simulink model "MohammadDBZ1"  (R2023b)
settings: Solver=ode15s  StartTime=0.0  StopTime=300  RelTol=1e-3
libraries: slpidlib x10
settings Model: PacingRate=10  Creator=Nezam Avaran  LastModifiedBy=Nezam Avaran

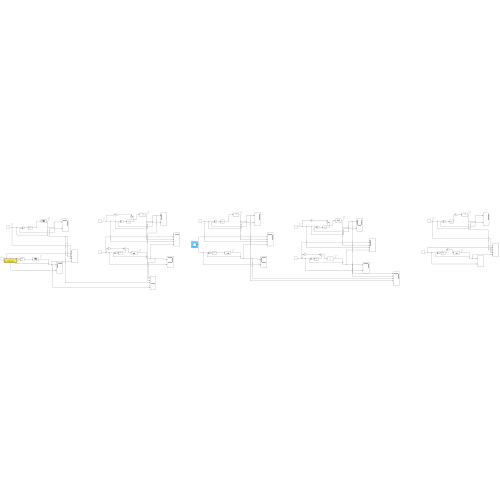
[thumbnail: Simulink's stored preview of the top-level diagram]
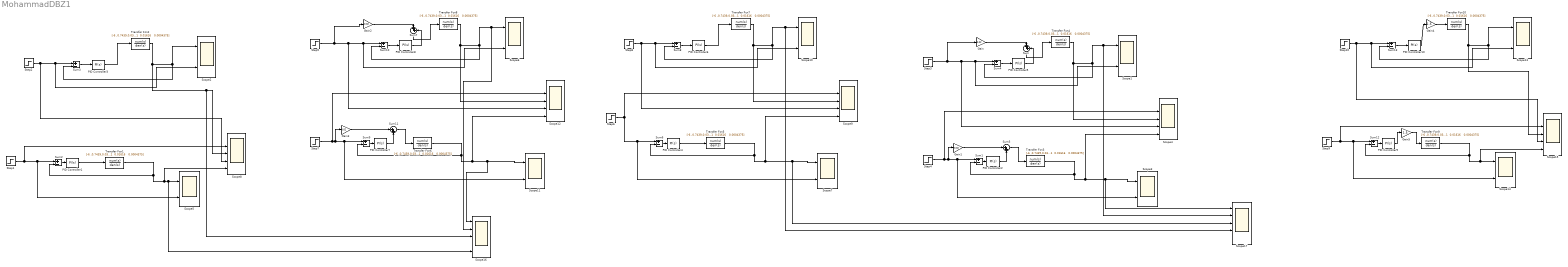
== system MohammadDBZ1 ==
  Gain{,1..3} (4 alike) : Gain  Gain=0.02
  Gain4 : Gain  Gain=1.5
  Gain5 : Gain  Gain=1.5
  PID Controller{1..2,4,7,9} (5 alike) : slpidlib/PID Controller  Controller=PI  Form=Ideal  TimeDomain=Continuous-time  UseExternalTs=off  SampleTime=-1  IntegratorMethod=Forward Euler  FilterMethod=Forward Euler  ControllerParametersSource=internal  P=0.00129745297341526  I=0.33499478649469  UseKiTs=off  D=0  N=100  UseFilter=on  TunerSelectOption=Transfer Function Based (PID Tuner App)  InitialConditionSource=internal  InitialConditionForIntegrator=0  InitialConditionForFilter=0  DifferentiatorICPrevScaledInput=0  ExternalReset=none  TrackingMode=off  Kt=1  LimitOutput=off  SatLimitsSource=internal  UpperSaturationLimit=inf  LowerSaturationLimit=-inf  LinearizeAsGain=on  AntiWindupMode=none  Kb=1  LimitIntegrator=off  UpperIntegratorSaturationLimit=inf  LowerIntegratorSaturationLimit=-inf  POutMin=[]  POutMax=[]  IOutMin=[]  IOutMax=[]  DOutMin=[]  DOutMax=[]  NOutMin=[]  NOutMax=[]  SumOutMin=[]  SumOutMax=[]  SaturationOutMin=[]  SaturationOutMax=[]  PParamMin=[]  PParamMax=[]  IParamMin=[]  IParamMax=[]  DParamMin=[]  DParamMax=[]  NParamMin=[]  NParamMax=[]  KbParamMin=[]  KbParamMax=[]  KtParamMin=[]  KtParamMax=[]  KbOutMin=[]  KbOutMax=[]  KtOutMin=[]  KtOutMax=[]  IntegratorOutMin=[]  IntegratorOutMax=[]  FilterOutMin=[]  FilterOutMax=[]  SumI1OutMin=[]  SumI1OutMax=[]  SumI2OutMin=[]  SumI2OutMax=[]  SumI3OutMin=[]  SumI3OutMax=[]  SumI4OutMin=[]  SumI4OutMax=[]  SumDOutMin=[]  SumDOutMax=[]  DifferentiatorOutMin=[]  DifferentiatorOutMax=[]  FilterDiffOutCoefMin=[]  FilterDiffOutCoefMax=[]  ReciprocalOutMin=[]  ReciprocalOutMax=[]  SumDenOutMin=[]  SumDenOutMax=[]  SumNumOutMin=[]  SumNumOutMax=[]  DivideOutMin=[]  DivideOutMax=[]  UdiffTsProdOutMin=[]  UdiffTsProdOutMax=[]  NTsProdOutMin=[]  NTsProdOutMax=[]  UintegralTsProdOutMin=[]  UintegralTsProdOutMax=[]  UngainTsProdOutMin=[]  UngainTsProdOutMax=[]  ClampingZeroOutDataTypeStr=Inherit: Inherit via back propagation  ClampingZeroOutMin=[]  ClampingZeroOutMax=[]  FilterDenConstantOutDataTypeStr=Inherit: Inherit via back propagation  FilterDenConstantOutMin=[]  FilterDenConstantOutMax=[]  PCopyOutDataTypeStr=Inherit: Inherit via back propagation  PCopyOutMin=[]  PCopyOutMax=[]  NCopyOutDataTypeStr=Inherit: Inherit via back propagation  NCopyOutMin=[]  NCopyOutMax=[]  IntegratorContinuousStateAttributes=''  IntegratorStateMustResolveToSignalObject=off  IntegratorRTWStateStorageClass=Auto  FilterContinuousStateAttributes=''  FilterStateMustResolveToSignalObject=off  FilterRTWStateStorageClass=Auto  ParallelPVariant=Passthrough  IdealPVariant=InternalParameters  IVariant=InternalParameters  DVariant=Disabled  IntegratorVariant=Continuous  SatVariant=Disabled  AWVariant=Passthrough  PCopyVariant=Disabled  TRVariant=Disabled  FdbkBlocksVariant=Forward  IdealPFdbkVariant=Disabled  SatFdbkVariant=Disabled  DerivativeFilterVariant=Disabled  NVariant=Disabled  NCopyVariant=Disabled_SignalSpec  FilterICVariant=Disabled  IntegratorICVariant=InternalICs  ExternalResetVariant=Disabled  TRSumVariant=Passthrough  SumFdbkVariant=Disabled  SumVariant=Sum_PI  TsampFilterVariant=InternalTs  TsampNgainVariant=Passthrough  TsampIntegralVariant=Disabled_SignalSpec  ExternalSaturationOutDataTypeStr=Inherit: Same as second input
  PID Controller{3,5..6,8,10} (5 alike) : slpidlib/PID Controller  Controller=PI  Form=Ideal  TimeDomain=Continuous-time  UseExternalTs=off  SampleTime=-1  IntegratorMethod=Forward Euler  FilterMethod=Forward Euler  ControllerParametersSource=internal  P=0.00251794980277336  I=0.176145493328416  UseKiTs=off  D=0  N=100  UseFilter=on  TunerSelectOption=Transfer Function Based (PID Tuner App)  InitialConditionSource=internal  InitialConditionForIntegrator=0  InitialConditionForFilter=0  DifferentiatorICPrevScaledInput=0  ExternalReset=none  TrackingMode=off  Kt=1  LimitOutput=off  SatLimitsSource=internal  UpperSaturationLimit=inf  LowerSaturationLimit=-inf  LinearizeAsGain=on  AntiWindupMode=none  Kb=1  LimitIntegrator=off  UpperIntegratorSaturationLimit=inf  LowerIntegratorSaturationLimit=-inf  POutMin=[]  POutMax=[]  IOutMin=[]  IOutMax=[]  DOutMin=[]  DOutMax=[]  NOutMin=[]  NOutMax=[]  SumOutMin=[]  SumOutMax=[]  SaturationOutMin=[]  SaturationOutMax=[]  PParamMin=[]  PParamMax=[]  IParamMin=[]  IParamMax=[]  DParamMin=[]  DParamMax=[]  NParamMin=[]  NParamMax=[]  KbParamMin=[]  KbParamMax=[]  KtParamMin=[]  KtParamMax=[]  KbOutMin=[]  KbOutMax=[]  KtOutMin=[]  KtOutMax=[]  IntegratorOutMin=[]  IntegratorOutMax=[]  FilterOutMin=[]  FilterOutMax=[]  SumI1OutMin=[]  SumI1OutMax=[]  SumI2OutMin=[]  SumI2OutMax=[]  SumI3OutMin=[]  SumI3OutMax=[]  SumI4OutMin=[]  SumI4OutMax=[]  SumDOutMin=[]  SumDOutMax=[]  DifferentiatorOutMin=[]  DifferentiatorOutMax=[]  FilterDiffOutCoefMin=[]  FilterDiffOutCoefMax=[]  ReciprocalOutMin=[]  ReciprocalOutMax=[]  SumDenOutMin=[]  SumDenOutMax=[]  SumNumOutMin=[]  SumNumOutMax=[]  DivideOutMin=[]  DivideOutMax=[]  UdiffTsProdOutMin=[]  UdiffTsProdOutMax=[]  NTsProdOutMin=[]  NTsProdOutMax=[]  UintegralTsProdOutMin=[]  UintegralTsProdOutMax=[]  UngainTsProdOutMin=[]  UngainTsProdOutMax=[]  ClampingZeroOutDataTypeStr=Inherit: Inherit via back propagation  ClampingZeroOutMin=[]  ClampingZeroOutMax=[]  FilterDenConstantOutDataTypeStr=Inherit: Inherit via back propagation  FilterDenConstantOutMin=[]  FilterDenConstantOutMax=[]  PCopyOutDataTypeStr=Inherit: Inherit via back propagation  PCopyOutMin=[]  PCopyOutMax=[]  NCopyOutDataTypeStr=Inherit: Inherit via back propagation  NCopyOutMin=[]  NCopyOutMax=[]  IntegratorContinuousStateAttributes=''  IntegratorStateMustResolveToSignalObject=off  IntegratorRTWStateStorageClass=Auto  FilterContinuousStateAttributes=''  FilterStateMustResolveToSignalObject=off  FilterRTWStateStorageClass=Auto  ParallelPVariant=Passthrough  IdealPVariant=InternalParameters  IVariant=InternalParameters  DVariant=Disabled  IntegratorVariant=Continuous  SatVariant=Disabled  AWVariant=Passthrough  PCopyVariant=Disabled  TRVariant=Disabled  FdbkBlocksVariant=Forward  IdealPFdbkVariant=Disabled  SatFdbkVariant=Disabled  DerivativeFilterVariant=Disabled  NVariant=Disabled  NCopyVariant=Disabled_SignalSpec  FilterICVariant=Disabled  IntegratorICVariant=InternalICs  ExternalResetVariant=Disabled  TRSumVariant=Passthrough  SumFdbkVariant=Disabled  SumVariant=Sum_PI  TsampFilterVariant=InternalTs  TsampNgainVariant=Passthrough  TsampIntegralVariant=Disabled_SignalSpec  ExternalSaturationOutDataTypeStr=Inherit: Same as second input
  Scope{1..3,5..7,10..11,13..14} (10 alike) : Scope  NumInputPorts=2
  Scope{4,8..9,12,15..17} (7 alike) : Scope  NumInputPorts=5
  Step1 : Step  Time=5  After=1.1*0.0389  SampleTime=0
  Step10 : Step  Time=5  After=0.9*0.0389  SampleTime=0
  Step2 : Step  Time=5  After=0.9*0.0389  SampleTime=0
  Step3 : Step  Time=5  After=0.9*20  SampleTime=0
  Step4 : Step  Time=5  After=1.1*20  SampleTime=0
  Step5 : Step  Time=5  After=0.9*0.0389  SampleTime=0
  Step6 : Step  Time=5  After=1.1*20  SampleTime=0
  Step7 : Step  Time=5  After=1.1*0.0389  SampleTime=0
  Step8 : Step  Time=5  After=0.9*20  SampleTime=0
  Step9 : Step  Time=5  After=1.1*0.0389  SampleTime=0
  Sum{,5,7,11} (4 alike) : Sum  Inputs=|++
  Sum{1..4,6,8..10,12..13} (10 alike) : Sum  Inputs=+-
  Transfer Fcn{1..10} (10 alike) : TransferFcn  Numerator=[-6 ,0.7439,0.03802]  Denominator="[1 0.1651  0.01616   0.0004375]"
  wires:
  Step6/1 -> Scope9/2, Sum6/1, Scope7/2
  PID Controller4/1 -> Transfer Fcn5/1
  Sum6/1 -> PID Controller4/1
  Transfer Fcn5/1 -> Sum6/2, Scope9/5, Scope17/3, Scope7/1
  PID Controller6/1 -> Transfer Fcn7/1
  Sum8/1 -> PID Controller6/1
  Transfer Fcn7/1 -> Scope9/3, Sum8/2, Scope17/4, Scope10/1
  Step8/1 -> Scope9/4, Sum8/1, Scope10/2
  Step2/1 -> Scope2/2, Sum3/1, Scope8/4
  Transfer Fcn2/1 -> Scope2/1, Sum3/2, Scope16/3, Scope8/3
  Sum3/1 -> PID Controller3/1
  PID Controller3/1 -> Transfer Fcn2/1
  Transfer Fcn1/1 -> Scope16/5, Scope5/1, Scope8/5, Sum2/2
  Sum2/1 -> PID Controller1/1
  PID Controller1/1 -> Transfer Fcn1/1
  Step1/1 -> Scope5/2, Sum2/1, Scope8/2
  Step3/1 -> Gain/1, Scope4/4, Scope1/2, Sum4/1
  Transfer Fcn4/1 -> Scope17/2, Scope1/1, Sum4/2, Scope4/3
  Sum4/1 -> PID Controller5/1
  PID Controller5/1 -> Sum/2
  Transfer Fcn3/1 -> Scope17/1, Scope3/1, Scope4/5, Sum1/2
  Sum1/1 -> PID Controller2/1
  PID Controller2/1 -> Sum5/2
  Step4/1 -> Scope4/2, Gain1/1, Scope3/2, Sum1/1
  Gain/1 -> Sum/1
  Sum/1 -> Transfer Fcn4/1
  Gain1/1 -> Sum5/1
  Sum5/1 -> Transfer Fcn3/1
  Sum11/1 -> Transfer Fcn6/1
  Sum9/1 -> PID Controller7/1
  Step5/1 -> Gain2/1, Scope12/4, Scope6/2, Sum10/1
  Sum10/1 -> PID Controller8/1
  Transfer Fcn8/1 -> Scope16/2, Scope6/1, Sum10/2, Scope12/3
  Gain2/1 -> Sum7/1
  PID Controller7/1 -> Sum11/2
  Transfer Fcn6/1 -> Scope16/1, Scope11/1, Scope12/5, Sum9/2
  Sum7/1 -> Transfer Fcn8/1
  PID Controller8/1 -> Sum7/2
  Step7/1 -> Scope12/2, Gain3/1, Scope11/2, Sum9/1
  Gain3/1 -> Sum11/1
  PID Controller9/1 -> Gain5/1
  Sum12/1 -> PID Controller9/1
  PID Controller10/1 -> Gain4/1
  Transfer Fcn9/1 -> Scope14/1, Scope15/5, Sum12/2
  Sum13/1 -> PID Controller10/1
  Step9/1 -> Scope14/2, Sum12/1, Scope15/2
  Step10/1 -> Scope13/2, Sum13/1, Scope15/4
  Transfer Fcn10/1 -> Scope13/1, Sum13/2, Scope15/3
  Gain4/1 -> Transfer Fcn10/1
  Gain5/1 -> Transfer Fcn9/1
